simulink model "beispiel"  (R2019b)
settings: Solver=VariableStepAuto  StartTime=0.0  StopTime=20  RelTol=1e-3
values from neighbouring files (symbols this model uses):
  a = 5    [beispielsystem.m]    (also in init_loesung.m = xdash0-xdash0*pp)
  b = 2    [beispielsystem.m]    (also in init.m = 0.8; init_loesung.m = xdash0+xdash0*pp; model_dsc.m = block.DialogPrm(3).data)
  Delta = 1    [beispielsystem.m]    (also in init.m; init_loesung.m = 0.01; model_dsc.m = block.DialogPrm(1).data)
settings Model: Creator=schauer  LastModifiedBy=schauer

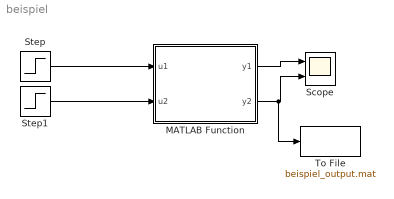
== system beispiel ==
  MATLAB Function : MATLAB Function  TreatAsAtomicUnit=on  SystemSampleTime=Delta
  Scope : Scope  NumInputPorts=2
  Step : Step  Time=5  Before=1  After=10  SampleTime=0
  Step1 : Step  Time=8  Before=-1  After=4  SampleTime=0
  To File : ToFile  Filename=beispiel_output.mat  MatrixName=y2_vec
  wires:
  Step1/1 -> MATLAB Function/2(u2)
  Step/1 -> MATLAB Function/1(u1)
  MATLAB Function/1(y1) -> Scope/1
  MATLAB Function/2(y2) -> To File/1, Scope/2

== matlab function beispiel/MATLAB Function ==
  data: u1 input; y1 output; u2 input; y2 output; a parameter; b parameter
function [y1,y2] = fcn(u1,u2,a, b)
%y1(k)=a*u1(k)+b*u2(k)
%y2(k)=max(y1(k))
%Delta=1s
%a und b sind Parameter, die über den Workspace definiert werden
%zu merken: max_y1 (last y2)
persistent y1_max;
if isempty(y1_max)
    y1_max=0;
end

y1=a*u1+b*u2;
y2=max(y1,y1_max);

y1_max=y2;
